simulink model "C28069_LLC_ePWM_V8_230307_PhaeShiftWorking"  (R2022b)
settings: Solver=FixedStepAuto  StartTime=0.0  StopTime=10  RelTol=1e-3  EnableMultiTasking=on
model workspace (MAT data in the model file):
  Comp_DAC = 512
undefined symbols (not defined in the file or in its folder): Down, GPTRIP1SEL, GPTRIP2SEL, PWM_Control, PWM_Gen, PWM_Gen1, SCI_A_Transmit, SCI_A_Transmit_Current_Suffix, SCI_A_Transmit_Duty_Suffix, SCI_A_Transmit_Freq_Suffix, SCI_A_Transmit_OVPFlag_Suffix, SCI_A_Transmit_PFC_Suffix, SCI_A_Transmit_SS_Suffix, SCI_A_Transmit_TBPHS_Suffix, SCI_A_Transmit_VADC_Suffix, SCI_A_Transmit_VAvg_Suffix, SCI_A_Transmit_VBAT_Suffix, SCI_A_Transmit_VBATRef_Suffix, SCI_A_Transmit_Vo_Suffix, TZ1, TZ2, u1, Up
libraries: c2802xlib x92, c280xlib x39, simulink x36, c2000lib x1
(part 4 of 18)

== system C28069_LLC_ePWM_V8_230307_PhaeShiftWorking/UART Reporting @ 1Hz/Send Current ==
  function : TriggerPort  TriggerType=function-call  VariantControl=(inherit)
  Data Store Read1 : DataStoreRead  DataStoreName=IoutCurrentBAT_Value  IndexOptions=Index vector (dialog)  Indices=1  OutputSizes=1
  Data Type Conversion : DataTypeConversion  OutDataTypeStr=double  SaturateOnIntegerOverflow=off  RndMeth=Floor
  Function Caller1 : FunctionCaller  FunctionPrototype=SCI_A_Transmit(u)  InputArgumentSpecifications=<Enter example>  OutputArgumentSpecifications=<Enter example>
  Function Caller2 : FunctionCaller  FunctionPrototype=SCI_A_Transmit_Current_Suffix()  InputArgumentSpecifications=<Enter example>  OutputArgumentSpecifications=<Enter example>
  wires:
  Data Type Conversion/1 -> Function Caller1/1
  Data Store Read1/1 -> Data Type Conversion/1

== system C28069_LLC_ePWM_V8_230307_PhaeShiftWorking/UART Reporting @ 1Hz/Send Duty ==
  function : TriggerPort  TriggerType=function-call  VariantControl=(inherit)
  Data Store Read1 : DataStoreRead  DataStoreName=Duty_Value  IndexOptions=Index vector (dialog)  Indices=1  OutputSizes=1
  Data Type Conversion : DataTypeConversion  OutDataTypeStr=double  SaturateOnIntegerOverflow=off  RndMeth=Floor
  Function Caller1 : FunctionCaller  FunctionPrototype=SCI_A_Transmit(u)  InputArgumentSpecifications=<Enter example>  OutputArgumentSpecifications=<Enter example>
  Function Caller2 : FunctionCaller  FunctionPrototype=SCI_A_Transmit_Duty_Suffix()  InputArgumentSpecifications=<Enter example>  OutputArgumentSpecifications=<Enter example>
  wires:
  Data Store Read1/1 -> Data Type Conversion/1
  Data Type Conversion/1 -> Function Caller1/1

== system C28069_LLC_ePWM_V8_230307_PhaeShiftWorking/UART Reporting @ 1Hz/Send Freq ==
  function : TriggerPort  TriggerType=function-call  VariantControl=(inherit)
  Data Store Read1 : DataStoreRead  DataStoreName=Freq_Value_Out  IndexOptions=Index vector (dialog)  Indices=1  OutputSizes=1
  Data Type Conversion : DataTypeConversion  OutDataTypeStr=double  SaturateOnIntegerOverflow=off  RndMeth=Floor
  Function Caller1 : FunctionCaller  FunctionPrototype=SCI_A_Transmit(u)  InputArgumentSpecifications=<Enter example>  OutputArgumentSpecifications=<Enter example>
  Function Caller2 : FunctionCaller  FunctionPrototype=SCI_A_Transmit_Freq_Suffix()  InputArgumentSpecifications=<Enter example>  OutputArgumentSpecifications=<Enter example>
  wires:
  Data Store Read1/1 -> Data Type Conversion/1
  Data Type Conversion/1 -> Function Caller1/1

== system C28069_LLC_ePWM_V8_230307_PhaeShiftWorking/UART Reporting @ 1Hz/Send OVPFlag ==
  function : TriggerPort  TriggerType=function-call  VariantControl=(inherit)
  Data Store Read1 : DataStoreRead  DataStoreName=OVP_Flag  IndexOptions=Index vector (dialog)  Indices=1  OutputSizes=1
  Data Type Conversion : DataTypeConversion  OutDataTypeStr=double  SaturateOnIntegerOverflow=off  RndMeth=Floor
  Function Caller1 : FunctionCaller  FunctionPrototype=SCI_A_Transmit(u)  InputArgumentSpecifications=<Enter example>  OutputArgumentSpecifications=<Enter example>
  Function Caller2 : FunctionCaller  FunctionPrototype=SCI_A_Transmit_OVPFlag_Suffix()  InputArgumentSpecifications=<Enter example>  OutputArgumentSpecifications=<Enter example>
  wires:
  Data Store Read1/1 -> Data Type Conversion/1
  Data Type Conversion/1 -> Function Caller1/1

== system C28069_LLC_ePWM_V8_230307_PhaeShiftWorking/UART Reporting @ 1Hz/Send PFC_OK ==
  function : TriggerPort  TriggerType=function-call  VariantControl=(inherit)
  Data Store Read1 : DataStoreRead  DataStoreName=PFC_OK  IndexOptions=Index vector (dialog)  Indices=1  OutputSizes=1
  Data Type Conversion : DataTypeConversion  OutDataTypeStr=double  SaturateOnIntegerOverflow=off  RndMeth=Floor
  Function Caller1 : FunctionCaller  FunctionPrototype=SCI_A_Transmit(u)  InputArgumentSpecifications=<Enter example>  OutputArgumentSpecifications=<Enter example>
  Function Caller2 : FunctionCaller  FunctionPrototype=SCI_A_Transmit_PFC_Suffix()  InputArgumentSpecifications=<Enter example>  OutputArgumentSpecifications=<Enter example>
  wires:
  Data Type Conversion/1 -> Function Caller1/1
  Data Store Read1/1 -> Data Type Conversion/1

== system C28069_LLC_ePWM_V8_230307_PhaeShiftWorking/UART Reporting @ 1Hz/Send SoftStart ==
  function : TriggerPort  TriggerType=function-call  VariantControl=(inherit)
  Data Store Read1 : DataStoreRead  DataStoreName=SoftStart_OK_Signal  IndexOptions=Index vector (dialog)  Indices=1  OutputSizes=1
  Data Type Conversion : DataTypeConversion  OutDataTypeStr=double  SaturateOnIntegerOverflow=off  RndMeth=Floor
  Function Caller1 : FunctionCaller  FunctionPrototype=SCI_A_Transmit(u)  InputArgumentSpecifications=<Enter example>  OutputArgumentSpecifications=<Enter example>
  Function Caller2 : FunctionCaller  FunctionPrototype=SCI_A_Transmit_SS_Suffix()  InputArgumentSpecifications=<Enter example>  OutputArgumentSpecifications=<Enter example>
  wires:
  Data Type Conversion/1 -> Function Caller1/1
  Data Store Read1/1 -> Data Type Conversion/1

== system C28069_LLC_ePWM_V8_230307_PhaeShiftWorking/UART Reporting @ 1Hz/Send TBPHS (PhaseShift) ==
  function : TriggerPort  TriggerType=function-call  VariantControl=(inherit)
  Data Store Read1 : DataStoreRead  DataStoreName=TBPHS  IndexOptions=Index vector (dialog)  Indices=1  OutputSizes=1
  Data Type Conversion : DataTypeConversion  OutDataTypeStr=double  SaturateOnIntegerOverflow=off  RndMeth=Floor
  Function Caller1 : FunctionCaller  FunctionPrototype=SCI_A_Transmit(u)  InputArgumentSpecifications=<Enter example>  OutputArgumentSpecifications=<Enter example>
  Function Caller2 : FunctionCaller  FunctionPrototype=SCI_A_Transmit_TBPHS_Suffix()  InputArgumentSpecifications=<Enter example>  OutputArgumentSpecifications=<Enter example>
  wires:
  Data Store Read1/1 -> Data Type Conversion/1
  Data Type Conversion/1 -> Function Caller1/1

== system C28069_LLC_ePWM_V8_230307_PhaeShiftWorking/UART Reporting @ 1Hz/Send VADC_Avg ==
  function : TriggerPort  TriggerType=function-call  VariantControl=(inherit)
  Data Store Read1 : DataStoreRead  DataStoreName=VBAT_ADC_AvgValue  IndexOptions=Index vector (dialog)  Indices=1  OutputSizes=1
  Data Type Conversion : DataTypeConversion  Commented=on  OutDataTypeStr=double  SaturateOnIntegerOverflow=off  RndMeth=Floor
  Function Caller1 : FunctionCaller  FunctionPrototype=SCI_A_Transmit(u)  InputArgumentSpecifications=<Enter example>  OutputArgumentSpecifications=<Enter example>
  Function Caller2 : FunctionCaller  FunctionPrototype=SCI_A_Transmit_VAvg_Suffix()  InputArgumentSpecifications=<Enter example>  OutputArgumentSpecifications=<Enter example>
  wires:
  Data Store Read1/1 -> Function Caller1/1

== system C28069_LLC_ePWM_V8_230307_PhaeShiftWorking/UART Reporting @ 1Hz/Send VBAT Value (Vout) ==
  function : TriggerPort  TriggerType=function-call  VariantControl=(inherit)
  Data Store Read1 : DataStoreRead  DataStoreName=VBAT_Value  IndexOptions=Index vector (dialog)  Indices=1  OutputSizes=1
  Data Type Conversion : DataTypeConversion  OutDataTypeStr=double  SaturateOnIntegerOverflow=off  RndMeth=Floor
  Function Caller1 : FunctionCaller  FunctionPrototype=SCI_A_Transmit(u)  InputArgumentSpecifications=<Enter example>  OutputArgumentSpecifications=<Enter example>
  Function Caller2 : FunctionCaller  FunctionPrototype=SCI_A_Transmit_VBAT_Suffix()  InputArgumentSpecifications=<Enter example>  OutputArgumentSpecifications=<Enter example>
  wires:
  Data Type Conversion/1 -> Function Caller1/1
  Data Store Read1/1 -> Data Type Conversion/1

== system C28069_LLC_ePWM_V8_230307_PhaeShiftWorking/UART Reporting @ 1Hz/Send VBAT Value (Vout)1 ==
  function : TriggerPort  TriggerType=function-call  VariantControl=(inherit)
  Data Store Read1 : DataStoreRead  DataStoreName=VBAT_Ref_Value  IndexOptions=Index vector (dialog)  Indices=1  OutputSizes=1
  Data Type Conversion : DataTypeConversion  OutDataTypeStr=double  SaturateOnIntegerOverflow=off  RndMeth=Floor
  Function Caller1 : FunctionCaller  FunctionPrototype=SCI_A_Transmit(u)  InputArgumentSpecifications=<Enter example>  OutputArgumentSpecifications=<Enter example>
  Function Caller2 : FunctionCaller  FunctionPrototype=SCI_A_Transmit_VBATRef_Suffix()  InputArgumentSpecifications=<Enter example>  OutputArgumentSpecifications=<Enter example>
  wires:
  Data Store Read1/1 -> Data Type Conversion/1
  Data Type Conversion/1 -> Function Caller1/1

== system C28069_LLC_ePWM_V8_230307_PhaeShiftWorking/UART Reporting @ 1Hz/Send Vo Value ==
  function : TriggerPort  TriggerType=function-call  VariantControl=(inherit)
  Data Store Read1 : DataStoreRead  DataStoreName=Vo_Value  IndexOptions=Index vector (dialog)  Indices=1  OutputSizes=1
  Data Type Conversion : DataTypeConversion  OutDataTypeStr=double  SaturateOnIntegerOverflow=off  RndMeth=Floor
  Function Caller1 : FunctionCaller  FunctionPrototype=SCI_A_Transmit(u)  InputArgumentSpecifications=<Enter example>  OutputArgumentSpecifications=<Enter example>
  Function Caller2 : FunctionCaller  FunctionPrototype=SCI_A_Transmit_Vo_Suffix()  InputArgumentSpecifications=<Enter example>  OutputArgumentSpecifications=<Enter example>
  wires:
  Data Store Read1/1 -> Data Type Conversion/1
  Data Type Conversion/1 -> Function Caller1/1

== system C28069_LLC_ePWM_V8_230307_PhaeShiftWorking/UART Reporting @ 1Hz/Send Voltage ADC Value ==
  function : TriggerPort  TriggerType=function-call  VariantControl=(inherit)
  Data Store Read1 : DataStoreRead  DataStoreName=VBAT_ADC_Value  IndexOptions=Index vector (dialog)  Indices=1  OutputSizes=1
  Data Type Conversion : DataTypeConversion  OutDataTypeStr=double  SaturateOnIntegerOverflow=off  RndMeth=Floor
  Function Caller1 : FunctionCaller  FunctionPrototype=SCI_A_Transmit(u)  InputArgumentSpecifications=<Enter example>  OutputArgumentSpecifications=<Enter example>
  Function Caller2 : FunctionCaller  FunctionPrototype=SCI_A_Transmit_VADC_Suffix()  InputArgumentSpecifications=<Enter example>  OutputArgumentSpecifications=<Enter example>
  wires:
  Data Store Read1/1 -> Data Type Conversion/1
  Data Type Conversion/1 -> Function Caller1/1

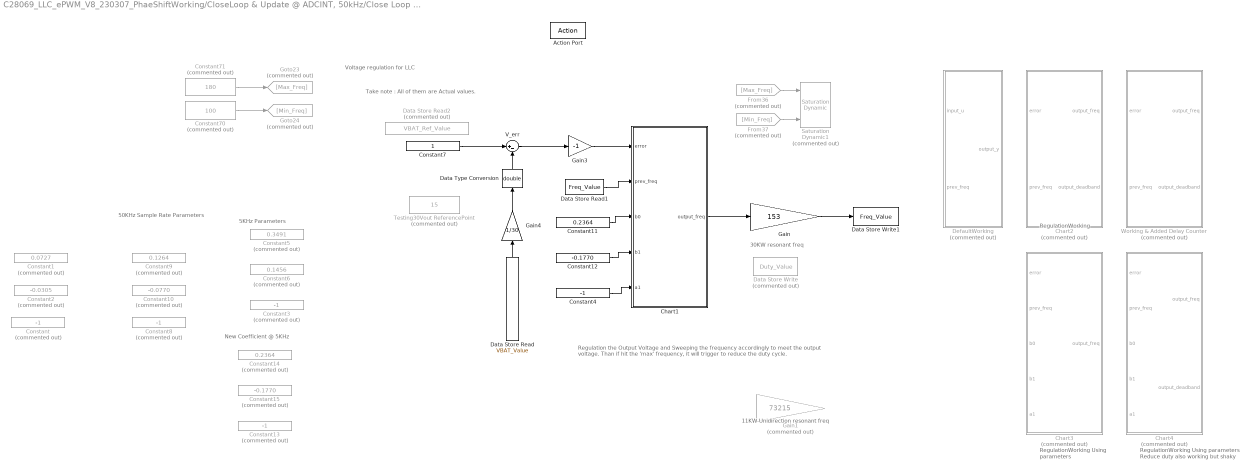
== system C28069_LLC_ePWM_V8_230307_PhaeShiftWorking/CloseLoop & Update @ ADCINT, 50kHz/Close Loop Regulation1/If Action Subsystem ==
  note: New Coefficient @ 5KHz
  note: 50KHz Sample Rate
      | Parameters
  note: RegulationWorking
  note: Regulation the Output Voltage and Sweeping the frequency accordingly to meet the output voltage.
      | Than if hit the 'max' frequency, it will trigger to reduce the duty cycle.
  note: Voltage regulation for LLC
  note: Take note : All of them are Actual values.
  note: 11KW Unidirection resonant freq
  note: 30KW resonant freq
  note: 5KHz Parameters
  note: RegulationWorking
      | Using parameters
  note: RegulationWorking
      | Using parameters
      | Reduce duty also working but shaky
  Action Port : ActionPort  ActionPortLabel=if((u1 == 1) & (u2 == 1))
  Chart1 : Stateflow chart  TreatAsAtomicUnit=on
  Chart2 : Stateflow chart  Commented=on  TreatAsAtomicUnit=on
  Chart3 : Stateflow chart  Commented=on  TreatAsAtomicUnit=on
  Chart4 : Stateflow chart  Commented=on  TreatAsAtomicUnit=on
  Constant{,3,8,13} (4 alike) : Constant  Commented=on  Value=-1  OutDataTypeStr=double
  Constant1 : Constant  Commented=on  Value=0.0727  OutDataTypeStr=double
  Constant10 : Constant  Commented=on  Value=-0.0770  OutDataTypeStr=double
  Constant11 : Constant  Value=0.2364  OutDataTypeStr=double
  Constant12 : Constant  Value=-0.1770  OutDataTypeStr=double
  Constant14 : Constant  Commented=on  Value=0.2364  OutDataTypeStr=double
  Constant15 : Constant  Commented=on  Value=-0.1770  OutDataTypeStr=double
  Constant2 : Constant  Commented=on  Value=-0.0305  OutDataTypeStr=double
  Constant4 : Constant  Value=-1  OutDataTypeStr=double
  Constant5 : Constant  Commented=on  Value=0.3491  OutDataTypeStr=double
  Constant6 : Constant  Commented=on  Value=0.1456  OutDataTypeStr=double
  Constant7 : Constant  OutDataTypeStr=double
  Constant70 : Constant  Commented=on  Value=100  OutDataTypeStr=double
  Constant71 : Constant  Commented=on  Value=180  OutDataTypeStr=double
  Constant9 : Constant  Commented=on  Value=0.1264  OutDataTypeStr=double
  Data Store Read : DataStoreRead  DataStoreName=VBAT_Value  IndexOptions=Index vector (dialog)  Indices=1  OutputSizes=1
  Data Store Read1 : DataStoreRead  DataStoreName=Freq_Value  IndexOptions=Index vector (dialog)  Indices=1  OutputSizes=1
  Data Store Read2 : DataStoreRead  Commented=on  DataStoreName=VBAT_Ref_Value  IndexOptions=Index vector (dialog)  Indices=1  OutputSizes=1
  Data Store Write : DataStoreWrite  Commented=on  DataStoreName=Duty_Value  IndexOptions=Index vector (dialog)  Indices=1  OutputSizes=1
  Data Store Write1 : DataStoreWrite  DataStoreName=Freq_Value  IndexOptions=Index vector (dialog)  Indices=1  OutputSizes=1
  Data Type Conversion : DataTypeConversion  OutDataTypeStr=double  SaturateOnIntegerOverflow=off  RndMeth=Floor
  DefaultWorking : Stateflow chart  Commented=on  TreatAsAtomicUnit=on
  From36 : From  Commented=on  GotoTag=Max_Freq
  From37 : From  Commented=on  GotoTag=Min_Freq
  Gain : Gain  Gain=153
  Gain1 : Gain  Commented=on  Gain=73215
  Gain3 : Gain  Gain=-1
  Gain4 : Gain  Gain=1/30
  Goto23 : Goto  Commented=on  GotoTag=Max_Freq
  Goto24 : Goto  Commented=on  GotoTag=Min_Freq
  Saturation Dynamic1 : simulink/Discontinuities/Saturation Dynamic  Commented=on  OutMin=[]  OutMax=[]  OutDataTypeStr=double  OutputDataTypeScalingMode=single  OutDataType=single  OutScaling=2^-10  DoSatur=off
  Testing30Vout ReferencePoint : Constant  Commented=on  Value=15  OutDataTypeStr=double
  V_err : Sum  Inputs=|+-  AccumDataTypeStr=double  OutDataTypeStr=double
  Working & Added Delay Counter : Stateflow chart  Commented=on  TreatAsAtomicUnit=on
  wires:
  Data Type Conversion/1 -> V_err/2
  Data Store Read1/1 -> Chart1/2(prev_freq)
  Constant70/1 -> Goto24/1
  From37/1 -> Saturation Dynamic1/3
  From36/1 -> Saturation Dynamic1/1
  V_err/1 -> Gain3/1
  Constant71/1 -> Goto23/1
  Chart1/1(output_freq) -> Gain/1
  Gain/1 -> Data Store Write1/1
  Data Store Read/1 -> Gain4/1
  Gain3/1 -> Chart1/1(error)
  Gain4/1 -> Data Type Conversion/1
  Constant11/1 -> Chart1/3(b0)
  Constant12/1 -> Chart1/4(b1)
  Constant4/1 -> Chart1/5(a1)
  Constant7/1 -> V_err/1

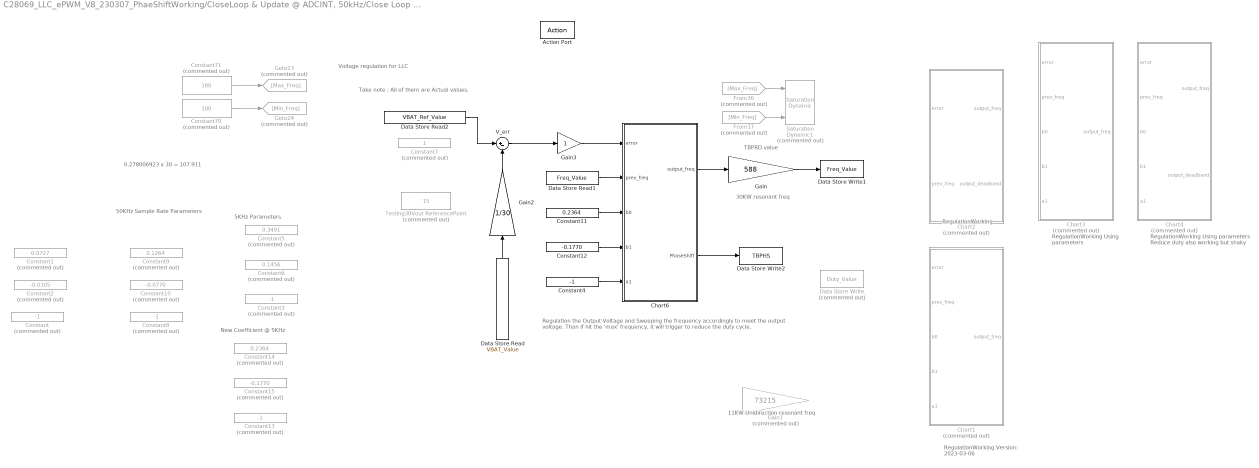
== system C28069_LLC_ePWM_V8_230307_PhaeShiftWorking/CloseLoop & Update @ ADCINT, 50kHz/Close Loop Regulation2/If Action Subsystem ==
  note: 0.278006923 x 30 = 107.911
  note: New Coefficient @ 5KHz
  note: 50KHz Sample Rate
      | Parameters
  note: RegulationWorking
  note: Regulation the Output Voltage and Sweeping the frequency accordingly to meet the output voltage.
      | Than if hit the 'max' frequency, it will trigger to reduce the duty cycle.
  note: Voltage regulation for LLC
  note: Take note : All of them are Actual values.
  note: 11KW Unidirection resonant freq
  note: 30KW resonant freq
  note: 5KHz Parameters
  note: RegulationWorking
      | Using parameters
  note: RegulationWorking
      | Using parameters
      | Reduce duty also working but shaky
  note: TBPRD value
  note: RegulationWorking
      | Version: 2023-03-06
  Action Port : ActionPort  ActionPortLabel=if((u1 == 1))
  Chart1 : Stateflow chart  Commented=on  TreatAsAtomicUnit=on
  Chart2 : Stateflow chart  Commented=on  TreatAsAtomicUnit=on
  Chart3 : Stateflow chart  Commented=on  TreatAsAtomicUnit=on
  Chart4 : Stateflow chart  Commented=on  TreatAsAtomicUnit=on
  Chart6 : Stateflow chart  TreatAsAtomicUnit=on
  Constant{,3,8,13} (4 alike) : Constant  Commented=on  Value=-1  OutDataTypeStr=double
  Constant1 : Constant  Commented=on  Value=0.0727  OutDataTypeStr=double
  Constant10 : Constant  Commented=on  Value=-0.0770  OutDataTypeStr=double
  Constant11 : Constant  Value=0.2364  OutDataTypeStr=double
  Constant12 : Constant  Value=-0.1770  OutDataTypeStr=double
  Constant14 : Constant  Commented=on  Value=0.2364  OutDataTypeStr=double
  Constant15 : Constant  Commented=on  Value=-0.1770  OutDataTypeStr=double
  Constant2 : Constant  Commented=on  Value=-0.0305  OutDataTypeStr=double
  Constant4 : Constant  Value=-1  OutDataTypeStr=double
  Constant5 : Constant  Commented=on  Value=0.3491  OutDataTypeStr=double
  Constant6 : Constant  Commented=on  Value=0.1456  OutDataTypeStr=double
  Constant7 : Constant  Commented=on  OutDataTypeStr=double
  Constant70 : Constant  Commented=on  Value=100  OutDataTypeStr=double
  Constant71 : Constant  Commented=on  Value=180  OutDataTypeStr=double
  Constant9 : Constant  Commented=on  Value=0.1264  OutDataTypeStr=double
  Data Store Read : DataStoreRead  DataStoreName=VBAT_Value  IndexOptions=Index vector (dialog)  Indices=1  OutputSizes=1
  Data Store Read1 : DataStoreRead  DataStoreName=Freq_Value  IndexOptions=Index vector (dialog)  Indices=1  OutputSizes=1
  Data Store Read2 : DataStoreRead  DataStoreName=VBAT_Ref_Value  IndexOptions=Index vector (dialog)  Indices=1  OutputSizes=1
  Data Store Write : DataStoreWrite  Commented=on  DataStoreName=Duty_Value  IndexOptions=Index vector (dialog)  Indices=1  OutputSizes=1
  Data Store Write1 : DataStoreWrite  DataStoreName=Freq_Value  IndexOptions=Index vector (dialog)  Indices=1  OutputSizes=1
  Data Store Write2 : DataStoreWrite  DataStoreName=TBPHS  IndexOptions=Index vector (dialog)  Indices=1  OutputSizes=1
  From36 : From  Commented=on  GotoTag=Max_Freq
  From37 : From  Commented=on  GotoTag=Min_Freq
  Gain : Gain  Gain=588
  Gain1 : Gain  Commented=on  Gain=73215
  Gain2 : Gain  Gain=1/30
  Gain3 : Gain
  Goto23 : Goto  Commented=on  GotoTag=Max_Freq
  Goto24 : Goto  Commented=on  GotoTag=Min_Freq
  Saturation Dynamic1 : simulink/Discontinuities/Saturation Dynamic  Commented=on  OutMin=[]  OutMax=[]  OutDataTypeStr=double  OutputDataTypeScalingMode=single  OutDataType=single  OutScaling=2^-10  DoSatur=off
  Testing30Vout ReferencePoint : Constant  Commented=on  Value=15  OutDataTypeStr=double
  V_err : Sum  Inputs=|+-  AccumDataTypeStr=double  OutDataTypeStr=double
  wires:
  Data Store Read1/1 -> Chart6/2(prev_freq)
  Constant70/1 -> Goto24/1
  From37/1 -> Saturation Dynamic1/3
  From36/1 -> Saturation Dynamic1/1
  V_err/1 -> Gain3/1
  Constant71/1 -> Goto23/1
  Gain/1 -> Data Store Write1/1
  Gain3/1 -> Chart6/1(error)
  Constant11/1 -> Chart6/3(b0)
  Constant12/1 -> Chart6/4(b1)
  Constant4/1 -> Chart6/5(a1)
  Data Store Read/1 -> Gain2/1
  Gain2/1 -> V_err/2
  Data Store Read2/1 -> V_err/1
  Chart6/1(output_freq) -> Gain/1
  Chart6/2(PhaseShift) -> Data Store Write2/1

== system C28069_LLC_ePWM_V8_230307_PhaeShiftWorking/CloseLoop & Update @ ADCINT, 50kHz/Control/Close Loop Regulation ==
  function : TriggerPort  TriggerType=function-call  VariantControl=(inherit)
  Constant : Constant
  Data Store Read1 : DataStoreRead  DataStoreName=SoftStart_OK_Signal  IndexOptions=Index vector (dialog)  Indices=1  OutputSizes=1
  Data Store Read4 : DataStoreRead  DataStoreName=PFC_OK  IndexOptions=Index vector (dialog)  Indices=1  OutputSizes=1
  If : If  NumInputs=2  IfExpression=(u1 == 1) & (u2 == 1)  ShowElse=off
  If Action Subsystem : Subsystem  TreatAsAtomicUnit=on
  wires:
  Constant/1 -> If/2
  If/1 -> If Action Subsystem/Action
  Data Store Read4/1 -> If/1

== system C28069_LLC_ePWM_V8_230307_PhaeShiftWorking/CloseLoop & Update @ ADCINT, 50kHz/Control/Debug ==
  function : TriggerPort  TriggerType=function-call  VariantControl=(inherit)
  Constant3 : Constant
  GPIO21 : c280xlib/Digital Output  GPIO_Number=GPIO16~GPIO23  GPIO_Bit0=off  GPIO_BIT0_Toggle=off  GPIO_Bit1=off  GPIO_BIT1_Toggle=off  GPIO_Bit2=off  GPIO_BIT2_Toggle=off  GPIO_Bit3=off  GPIO_BIT3_Toggle=off  GPIO_Bit4=off  GPIO_BIT4_Toggle=off  GPIO_Bit5=on  GPIO_BIT5_Toggle=off  GPIO_Bit6=off  GPIO_BIT6_Toggle=off  GPIO_Bit7=off  GPIO_BIT7_Toggle=off
  wires:
  Constant3/1 -> GPIO21/1

== system C28069_LLC_ePWM_V8_230307_PhaeShiftWorking/CloseLoop & Update @ ADCINT, 50kHz/Control/Debug1 ==
  function : TriggerPort  TriggerType=function-call  VariantControl=(inherit)
  Constant3 : Constant  Value=0
  GPIO21 : c280xlib/Digital Output  GPIO_Number=GPIO16~GPIO23  GPIO_Bit0=off  GPIO_BIT0_Toggle=off  GPIO_Bit1=off  GPIO_BIT1_Toggle=off  GPIO_Bit2=off  GPIO_BIT2_Toggle=off  GPIO_Bit3=off  GPIO_BIT3_Toggle=off  GPIO_Bit4=off  GPIO_BIT4_Toggle=off  GPIO_Bit5=on  GPIO_BIT5_Toggle=off  GPIO_Bit6=off  GPIO_BIT6_Toggle=off  GPIO_Bit7=off  GPIO_BIT7_Toggle=off
  wires:
  Constant3/1 -> GPIO21/1

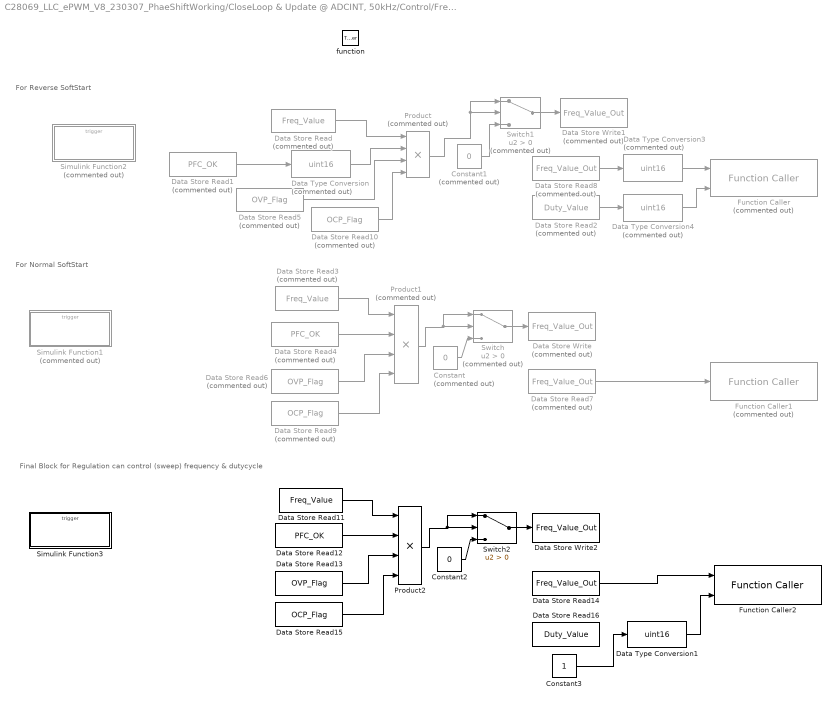
== system C28069_LLC_ePWM_V8_230307_PhaeShiftWorking/CloseLoop & Update @ ADCINT, 50kHz/Control/Frequency Update ==
  note: For Reverse SoftStart
  note: For Normal SoftStart
  note: Final Block for Regulation can control (sweep) frequency & dutycycle
  function : TriggerPort  TriggerType=function-call  VariantControl=(inherit)
  Constant : Constant  Commented=on  Value=0  OutDataTypeStr=double
  Constant1 : Constant  Commented=on  Value=0
  Constant2 : Constant  Value=0  OutDataTypeStr=double
  Constant3 : Constant  OutDataTypeStr=double
  Data Store Read : DataStoreRead  Commented=on  DataStoreName=Freq_Value  IndexOptions=Index vector (dialog)  Indices=1  OutputSizes=1
  Data Store Read1 : DataStoreRead  Commented=on  DataStoreName=PFC_OK  IndexOptions=Index vector (dialog)  Indices=1  OutputSizes=1
  Data Store Read10 : DataStoreRead  Commented=on  DataStoreName=OCP_Flag  IndexOptions=Index vector (dialog)  Indices=1  OutputSizes=1
  Data Store Read11 : DataStoreRead  DataStoreName=Freq_Value  IndexOptions=Index vector (dialog)  Indices=1  OutputSizes=1
  Data Store Read12 : DataStoreRead  DataStoreName=PFC_OK  IndexOptions=Index vector (dialog)  Indices=1  OutputSizes=1
  Data Store Read13 : DataStoreRead  DataStoreName=OVP_Flag  IndexOptions=Index vector (dialog)  Indices=1  OutputSizes=1
  Data Store Read14 : DataStoreRead  DataStoreName=Freq_Value_Out  IndexOptions=Index vector (dialog)  Indices=1  OutputSizes=1
  Data Store Read15 : DataStoreRead  DataStoreName=OCP_Flag  IndexOptions=Index vector (dialog)  Indices=1  OutputSizes=1
  Data Store Read16 : DataStoreRead  DataStoreName=Duty_Value  IndexOptions=Index vector (dialog)  Indices=1  OutputSizes=1
  Data Store Read2 : DataStoreRead  Commented=on  DataStoreName=Duty_Value  IndexOptions=Index vector (dialog)  Indices=1  OutputSizes=1
  Data Store Read3 : DataStoreRead  Commented=on  DataStoreName=Freq_Value  IndexOptions=Index vector (dialog)  Indices=1  OutputSizes=1
  Data Store Read4 : DataStoreRead  Commented=on  DataStoreName=PFC_OK  IndexOptions=Index vector (dialog)  Indices=1  OutputSizes=1
  Data Store Read5 : DataStoreRead  Commented=on  DataStoreName=OVP_Flag  IndexOptions=Index vector (dialog)  Indices=1  OutputSizes=1
  Data Store Read6 : DataStoreRead  Commented=on  DataStoreName=OVP_Flag  IndexOptions=Index vector (dialog)  Indices=1  OutputSizes=1
  Data Store Read7 : DataStoreRead  Commented=on  DataStoreName=Freq_Value_Out  IndexOptions=Index vector (dialog)  Indices=1  OutputSizes=1
  Data Store Read8 : DataStoreRead  Commented=on  DataStoreName=Freq_Value_Out  IndexOptions=Index vector (dialog)  Indices=1  OutputSizes=1
  Data Store Read9 : DataStoreRead  Commented=on  DataStoreName=OCP_Flag  IndexOptions=Index vector (dialog)  Indices=1  OutputSizes=1
  Data Store Write : DataStoreWrite  Commented=on  DataStoreName=Freq_Value_Out  IndexOptions=Index vector (dialog)  Indices=1  OutputSizes=1
  Data Store Write1 : DataStoreWrite  Commented=on  DataStoreName=Freq_Value_Out  IndexOptions=Index vector (dialog)  Indices=1  OutputSizes=1
  Data Store Write2 : DataStoreWrite  DataStoreName=Freq_Value_Out  IndexOptions=Index vector (dialog)  Indices=1  OutputSizes=1
  Data Type Conversion : DataTypeConversion  Commented=on  OutDataTypeStr=uint16  SaturateOnIntegerOverflow=off  RndMeth=Floor
  Data Type Conversion1 : DataTypeConversion  OutDataTypeStr=uint16  SaturateOnIntegerOverflow=off  RndMeth=Floor
  Data Type Conversion3 : DataTypeConversion  Commented=on  OutDataTypeStr=uint16  SaturateOnIntegerOverflow=off  RndMeth=Floor
  Data Type Conversion4 : DataTypeConversion  Commented=on  OutDataTypeStr=uint16  SaturateOnIntegerOverflow=off  RndMeth=Floor
  Function Caller : FunctionCaller  Commented=on  FunctionPrototype=PWM_Gen1(u,u1)  InputArgumentSpecifications=<Enter example>  OutputArgumentSpecifications=<Enter example>
  Function Caller1 : FunctionCaller  Commented=on  FunctionPrototype=PWM_Gen(u)  InputArgumentSpecifications=<Enter example>  OutputArgumentSpecifications=<Enter example>
  Function Caller2 : FunctionCaller  FunctionPrototype=PWM_Control(u,u1)  InputArgumentSpecifications=<Enter example>  OutputArgumentSpecifications=<Enter example>
  Product : Product  Commented=on  Inputs=4  OutDataTypeStr=uint16
  Product1 : Product  Commented=on  Inputs=4  OutDataTypeStr=double
  Product2 : Product  Inputs=4  OutDataTypeStr=double
  Simulink Function1 : Subsystem  Commented=on  TreatAsAtomicUnit=on
  Simulink Function2 : Subsystem  Commented=on  TreatAsAtomicUnit=on
  Simulink Function3 : Subsystem  TreatAsAtomicUnit=on
  Switch : Switch  Commented=on  Criteria=u2 > Threshold  OutDataTypeStr=double  SaturateOnIntegerOverflow=off  InputSameDT=off
  Switch1 : Switch  Commented=on  Criteria=u2 > Threshold  SaturateOnIntegerOverflow=off  InputSameDT=off
  Switch2 : Switch  Criteria=u2 > Threshold  OutDataTypeStr=double  SaturateOnIntegerOverflow=off  InputSameDT=off
  wires:
  Data Store Read1/1 -> Data Type Conversion/1
  Data Type Conversion/1 -> Product/2
  Data Store Read7/1 -> Function Caller1/1
  Product1/1 -> Switch/2, Switch/1
  Data Store Read2/1 -> Data Type Conversion4/1
  Data Store Read10/1 -> Product/4
  Data Store Read5/1 -> Product/3
  Constant1/1 -> Switch1/3
  Data Store Read4/1 -> Product1/2
  Data Store Read/1 -> Product/1
  Product/1 -> Switch1/2, Switch1/1
  Data Store Read9/1 -> Product1/4
  Constant/1 -> Switch/3
  Data Type Conversion3/1 -> Function Caller/1
  Data Store Read6/1 -> Product1/3
  Switch1/1 -> Data Store Write1/1
  Switch/1 -> Data Store Write/1
  Data Type Conversion4/1 -> Function Caller/2
  Data Store Read3/1 -> Product1/1
  Data Store Read8/1 -> Data Type Conversion3/1
  Constant2/1 -> Switch2/3
  Data Store Read11/1 -> Product2/1
  Switch2/1 -> Data Store Write2/1
  Data Store Read15/1 -> Product2/4
  Data Store Read13/1 -> Product2/3
  Product2/1 -> Switch2/2, Switch2/1
  Data Store Read12/1 -> Product2/2
  Data Store Read14/1 -> Function Caller2/1
  Data Type Conversion1/1 -> Function Caller2/2
  Constant3/1 -> Data Type Conversion1/1

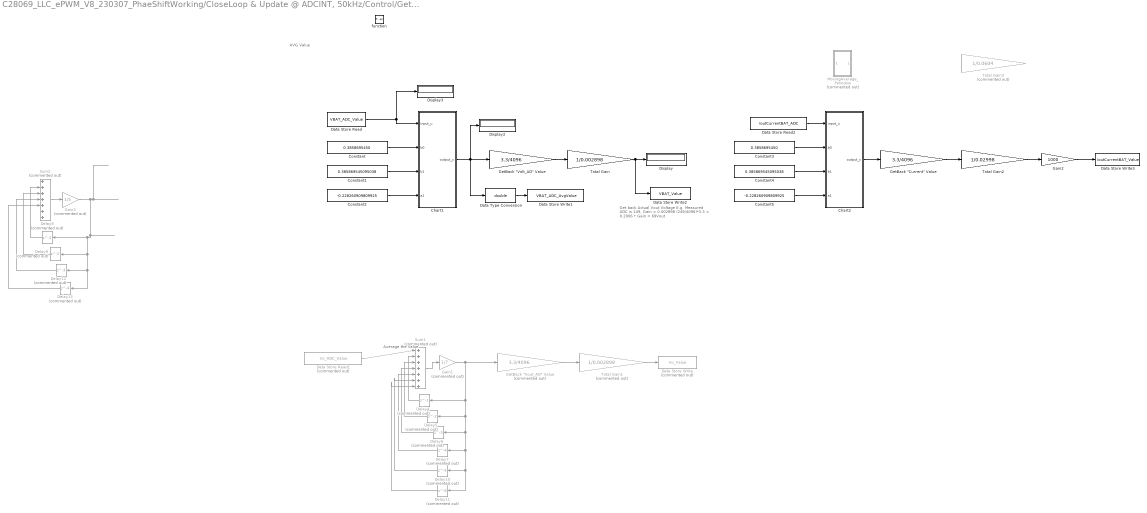
== system C28069_LLC_ePWM_V8_230307_PhaeShiftWorking/CloseLoop & Update @ ADCINT, 50kHz/Control/Get AVG2 ==
  note: AVG Value
  note: Average the value
  note: Get back Actual Vout Voltage
      | E.g.
      | Measured ADC is 249, Gain = 0.002898
      | (249/4096)*3.3 = 0.2006 * Gain
      | = 69Vout
  function : TriggerPort  TriggerType=function-call  VariantControl=(inherit)
  Chart1 : Stateflow chart  TreatAsAtomicUnit=on
  Chart2 : Stateflow chart  TreatAsAtomicUnit=on
  Constant : Constant  Value=0.3858695450
  Constant1 : Constant  Value=0.385869545095038
  Constant2 : Constant  Value=-0.228260909809925
  Constant3 : Constant  Value=0.3858695450
  Constant4 : Constant  Value=0.385869545095038
  Constant5 : Constant  Value=-0.228260909809925
  Data Store Read : DataStoreRead  DataStoreName=VBAT_ADC_Value  IndexOptions=Index vector (dialog)  Indices=1  OutputSizes=1
  Data Store Read1 : DataStoreRead  Commented=on  DataStoreName=Vo_ADC_Value  IndexOptions=Index vector (dialog)  Indices=1  OutputSizes=1
  Data Store Read2 : DataStoreRead  DataStoreName=IoutCurrentBAT_ADC  IndexOptions=Index vector (dialog)  Indices=1  OutputSizes=1
  Data Store Write : DataStoreWrite  Commented=on  DataStoreName=Vo_Value  IndexOptions=Index vector (dialog)  Indices=1  OutputSizes=1
  Data Store Write1 : DataStoreWrite  DataStoreName=VBAT_ADC_AvgValue  IndexOptions=Index vector (dialog)  Indices=1  OutputSizes=1
  Data Store Write2 : DataStoreWrite  DataStoreName=VBAT_Value  IndexOptions=Index vector (dialog)  Indices=1  OutputSizes=1
  Data Store Write3 : DataStoreWrite  DataStoreName=IoutCurrentBAT_Value  IndexOptions=Index vector (dialog)  Indices=1  OutputSizes=1
  Data Type Conversion : DataTypeConversion  OutDataTypeStr=double  SaturateOnIntegerOverflow=off  RndMeth=Floor
  Delay10 : Delay  Commented=on  DelayLength=5
  Delay11 : Delay  Commented=on  DelayLength=6
  Delay12 : Delay  Commented=on  DelayLength=3
  Delay13 : Delay  Commented=on  DelayLength=4
  Delay4 : Delay  Commented=on  DelayLength=1
  Delay5 : Delay  Commented=on
  Delay6 : Delay  Commented=on  DelayLength=3
  Delay7 : Delay  Commented=on  DelayLength=4
  Delay8 : Delay  Commented=on  DelayLength=1
  Delay9 : Delay  Commented=on
  Display : Display
      settings: Decimation=2
  Display2 : Display
  Display3 : Display
  Gain1 : Gain  Commented=on  Gain=1/7  OutDataTypeStr=uint16
  Gain2 : Gain  Gain=1000
  Gain3 : Gain  Commented=on  Gain=1/5  OutDataTypeStr=uint16
  "GetBack \"Current\" Value" : Gain  Gain=3.3/4096  OutDataTypeStr=double
  "GetBack \"Volt_AD\" Value" : Gain  Gain=3.3/4096  OutDataTypeStr=double
  "GetBack \"Vout_AD\" Value" : Gain  Commented=on  Gain=3.3/4096  OutDataTypeStr=double
  MovingAverage_7Window : Subsystem  Commented=on
  Sum1 : Sum  Commented=on  Inputs=|+++++++
  Sum2 : Sum  Commented=on  Inputs=|+++++++
  Total Gain : Gain  Gain=1/0.002898  OutDataTypeStr=double
  Total Gain1 : Gain  Commented=on  Gain=1/0.002898  OutDataTypeStr=double
  Total Gain2 : Gain  Gain=1/0.02998  OutDataTypeStr=double
  Total Gain3 : Gain  Commented=on  Gain=1/0.0604  OutDataTypeStr=double
  wires:
  Delay4/1 -> Sum1/2
  Total Gain1/1 -> Data Store Write/1
  "GetBack \"Current\" Value"/1 -> Total Gain2/1
  Delay7/1 -> Sum1/5
  Gain1/1 -> Delay4/1, Delay5/1, Delay6/1, Delay7/1, Delay10/1, Delay11/1, "GetBack \"Vout_AD\" Value"/1
  Data Type Conversion/1 -> Data Store Write1/1
  Delay6/1 -> Sum1/4
  Delay11/1 -> Sum1/7
  Delay10/1 -> Sum1/6
  "GetBack \"Vout_AD\" Value"/1 -> Total Gain1/1
  "GetBack \"Volt_AD\" Value"/1 -> Total Gain/1
  Data Store Read1/1 -> Sum1/1
  Total Gain/1 -> Display/1, Data Store Write2/1
  Sum1/1 -> Gain1/1
  Delay5/1 -> Sum1/3
  Total Gain2/1 -> Gain2/1
  Gain2/1 -> Data Store Write3/1
  Gain3/1 -> Delay9/1, Delay12/1, Delay13/1, Delay8/1
  Delay9/1 -> Sum2/3
  Sum2/1 -> Gain3/1
  Delay13/1 -> Sum2/5
  Delay12/1 -> Sum2/4
  Delay8/1 -> Sum2/2
  Data Store Read/1 -> Chart1/1(input_u), Display3/1
  Constant2/1 -> Chart1/4(a1)
  Constant1/1 -> Chart1/3(b1)
  Constant/1 -> Chart1/2(b0)
  Chart1/1(output_y) -> Display2/1, Data Type Conversion/1, "GetBack \"Volt_AD\" Value"/1
  Constant3/1 -> Chart2/2(b0)
  Constant4/1 -> Chart2/3(b1)
  Constant5/1 -> Chart2/4(a1)
  Data Store Read2/1 -> Chart2/1(input_u)
  Chart2/1(output_y) -> "GetBack \"Current\" Value"/1

== system C28069_LLC_ePWM_V8_230307_PhaeShiftWorking/CloseLoop & Update @ ADCINT, 50kHz/Frequency Update/Simulink Function1 ==
  note: Original
  note: Frequency Input Selection
  note: Control CMPA/B to Zero
      | When the input is <1KHz
      | (To switch off ePWM)
  note: Fixing deadtime to 250ns
  note: Added Trigger
  note: For F28069M
  PWM_Control2 : TriggerPort  TriggerType=function-call  IsSimulinkFunction=on  FunctionName=PWM_Control2  FunctionVisibility=scoped  VariantControl=(inherit)
  CMPA : Display
  CMPA1 : Display
  CMPB : Display
  CMPB1 : Display
  Constant : Constant  Value=100
  Constant1 : Constant
  Constant2 : Constant  Value=0
  Constant3 : Constant  Commented=on  Value=50
  Constant4 : Constant
  Dead time (%) : Display
  Dead time (sec) : Constant  Value=250E-9
  Divide : Product  Inputs=*/
  Floor : Rounding
  Gain : Gain  Gain=1/45000
  Gain1 : Gain  Gain=1000
  Gain2 : Gain  Gain=100
  Product1 : Product  Inputs=3
  Product2 : Product
  Product3 : Product
  Product4 : Product
  Subsystem1 : Subsystem  Commented=on
  Subtract : Sum  Inputs=+-
  Switch : Switch  Criteria=u2 > Threshold  Threshold=1  SaturateOnIntegerOverflow=off  InputSameDT=off
  Switch1 : Switch  Criteria=u2 > Threshold  OutDataTypeStr=double  SaturateOnIntegerOverflow=off  InputSameDT=off
  ePWM1 : c2802xlib/ePWM  PwmType=C2000  useModule=ePWM6  ePWMxLINKTBPRD=Not Linked  periodUnits=Clock cycles  timerSource=Input port  timerPeriod_clk=294  timerPeriod_sec=0.0001  tbshadow=Counter equals to zero  countingMode=Up-Down  phaseActiveEnable=Disable  phaseDirection=Count down after sync  phaseActive=0  synchronizationEnable=off  dcaevt1Sync=off  dcbevt1Sync=off  synchronizationOption=Disable  dcbevt1SyncOut=off  dcaevt1SyncOut=off  cmpdSyncOut=off  cmpcSyncOut=off  cmpbSyncOut=off  zeroSyncOut=off  swfSyncOut=off  perSynchronizationOption=Counter equals to period (CTR=PRD)  clockPrescale=1  HSclockPrescale=1  enswap=off  ePWMxAStatus=on  ePWMxAactionLogic1=Do nothing  ePWMxAactionLogic2=Do nothing  ePWMxAactionLogic3=Set  ePWMxAactionLogic4=Do nothing  ePWMxAactionLogic5=Clear  ePWMxAactionLogic6=Do nothing  ePWMxACSFenable=off  ePWMxACSFvalue=Forcing disable  ePWMxASFreload=Zero  ePWMxBStatus=on  ePWMxBactionLogic1=Do nothing  ePWMxBactionLogic2=Do nothing  ePWMxBactionLogic3=Do nothing  ePWMxBactionLogic4=Clear  ePWMxBactionLogic5=Do nothing  ePWMxBactionLogic6=Set  ePWMxBCSFenable=off  ePWMxBCSFvalue=Forcing disable  ePWMxBSFreload=Zero  ePWNxBOutWay=off  ePWMxLINKCMPA=Not Linked  CMPAUnits=Clock cycles  CMPASource=Input port  CMPAValue_per=50  CMPAValue_clk=0  enCMPAshadow=Counter equals to zero (CTR=Zero)  ePWMxLINKCMPB=Not Linked  CMPBUnits=Clock cycles  CMPBSource=Input port  CMPBValue_per=50  CMPBValue_clk=0  enCMPBshadow=Counter equals to zero (CTR=Zero)  ePWMxLINKCMPC=Not Linked  CMPCUnits=Clock cycles  CMPCSource=Specify via dialog  CMPCValue_per=50  CMPCValue_clk=32000  enCMPCshadow=Counter equals to zero (CTR=Zero)  ePWMxLINKCMPD=Not Linked  CMPDUnits=Clock cycles  CMPDSource=Specify via dialog  CMPDValue_per=50  CMPDValue_clk=32000  enCMPDshadow=Counter equals to zero (CTR=Zero)  enableDBePWMxA=off  enableDBePWMxB=off  enhalfcycle=off  DBpolarity=Active high complementary (AHC)  DBedgeDelay=Positive  DBSource_ePWMxA=ePWMxA  DBSource_ePWMxB=ePWMxA  DBPeriodUnits=Clock cycles  DBperiodSource=Input port  REDperiod=10  FEDperiod=10  REDperiod_sec=0  FEDperiod_sec=0  LoadModeDBRED=Immediate without using shadow  LoadModeDBFED=Immediate without using shadow  adcstartModuleA=off  adcrequestEventA=First event  adcstartEventA=Counter equals to zero (CTR=Zero)  adcstartEventA_type2=Digital Compare Module A Event 1 start of conversion (DCAEVT1.soc)  adcstartModuleB=off  adcrequestEventB=First event  adcstartEventB=Counter equals to zero (CTR=Zero)  adcstartEventB_type2=Counter equals to zero (CTR=Zero)  intEn=off  intPrd=First event  intSel=Counter equals to zero (CTR=Zero)  intSel_type2=Counter equals to zero (CTR=Zero)  hrpe=off  enHRPWM=off  HRPWM_LoadMode=Counter equals to period (CTR=PRD)  HRPWM_CTLMode=Duty or Period control mode  HRPWM_EDGMode=Both edge  hrpeb=off  enHRPWMB=off  HRPWM_LoadModeB=Counter equals to zero (CTR=ZERO)  HRPWM_CTLModeB=Duty or Period control mode  HRPWM_EDGModeB=Both edge  enHRDBRED=off  enHRDBFED=off  enSFO=on  enautoconv=on  chopperEnable=off  chopperFrequency=1  chopperFirstwidth=1  chopperDuty=12.5%  tripZonesource=Specify via dialog  tzselOSHT1=off  tzselOSHT2=off  tzselOSHT3=off  tzselOSHDCAEV1=off  tzselOSHDCBEV1=off  tzselCBC1=off  tzselCBC2=off  tzselCBC3=off  tzselCBCDCAEV2=off  tzselCBCDCBEV2=off  tzselOSHT4=off  tzselOSHT5=off  tzselOSHT6=off  tzselCBC4=off  tzselCBC5=off  tzselCBC6=off  enTzOstIntr=off  enTzCbcIntr=off  enTzDCAEVT1Intr=off  enTzDCAEVT2Intr=off  enTzDCBEVT1Intr=off  enTzDCBEVT2Intr=off  ePWMxAforced=No action  ePWMxBforced=No action  DCAEVT1forced=Low  DCBEVT1forced=Low  DCAEVT2forced=No action  DCBEVT2forced=No action  dcah=COMP1OUT input  dcal=Trip Zone 1 input (TZ1)  dcbh=COMP1OUT input  dcbl=Trip Zone 1 input (TZ1)  dcah_type2=GPTRIP1SEL/(TZ1)  dcal_type2=GPTRIP2SEL/(TZ2)  dcbh_type2=GPTRIP1SEL/(TZ1)  dcbl_type2=GPTRIP2SEL/(TZ2)  gendcaevt1=DCAH=high and DCAL=don't care  gendcaevt2=Event disabled  gendcbevt1=DCBH=high and DCBL=don't care  gendcbevt2=Event disabled  dcaevt1src=DCAEVT1 with sync  dcaevt2src=DCAEVT2 with sync  dcbevt1src=DCBEVT1 with sync  dcbevt2src=DCBEVT2 with sync  pulsesel=Counter equals to zero (CTR=Zero)  blankinv=off  blankoffset=0  blankwidth=0  evsrcsel=Filtered version of DCAEVT1 (DCAEVT1FILT)  encape=off
      settings: LibrarySourceBlock=c2806xlib/ePWM
  ePWM4 : c2802xlib/ePWM  PwmType=C2000  useModule=ePWM5  ePWMxLINKTBPRD=Not Linked  periodUnits=Clock cycles  timerSource=Input port  timerPeriod_clk=294  timerPeriod_sec=0.0001  tbshadow=Counter equals to zero  countingMode=Up-Down  phaseActiveEnable=Disable  phaseDirection=Count down after sync  phaseActive=0  synchronizationEnable=off  dcaevt1Sync=off  dcbevt1Sync=off  synchronizationOption=Disable  dcbevt1SyncOut=off  dcaevt1SyncOut=off  cmpdSyncOut=off  cmpcSyncOut=off  cmpbSyncOut=off  zeroSyncOut=off  swfSyncOut=off  perSynchronizationOption=Counter equals to period (CTR=PRD)  clockPrescale=1  HSclockPrescale=1  enswap=off  ePWMxAStatus=on  ePWMxAactionLogic1=Do nothing  ePWMxAactionLogic2=Do nothing  ePWMxAactionLogic3=Set  ePWMxAactionLogic4=Do nothing  ePWMxAactionLogic5=Clear  ePWMxAactionLogic6=Do nothing  ePWMxACSFenable=off  ePWMxACSFvalue=Forcing disable  ePWMxASFreload=Zero  ePWMxBStatus=on  ePWMxBactionLogic1=Do nothing  ePWMxBactionLogic2=Do nothing  ePWMxBactionLogic3=Do nothing  ePWMxBactionLogic4=Clear  ePWMxBactionLogic5=Do nothing  ePWMxBactionLogic6=Set  ePWMxBCSFenable=off  ePWMxBCSFvalue=Forcing disable  ePWMxBSFreload=Zero  ePWNxBOutWay=off  ePWMxLINKCMPA=Not Linked  CMPAUnits=Clock cycles  CMPASource=Input port  CMPAValue_per=50  CMPAValue_clk=0  enCMPAshadow=Counter equals to zero (CTR=Zero)  ePWMxLINKCMPB=Not Linked  CMPBUnits=Clock cycles  CMPBSource=Input port  CMPBValue_per=50  CMPBValue_clk=0  enCMPBshadow=Counter equals to zero (CTR=Zero)  ePWMxLINKCMPC=Not Linked  CMPCUnits=Clock cycles  CMPCSource=Specify via dialog  CMPCValue_per=50  CMPCValue_clk=32000  enCMPCshadow=Counter equals to zero (CTR=Zero)  ePWMxLINKCMPD=Not Linked  CMPDUnits=Clock cycles  CMPDSource=Specify via dialog  CMPDValue_per=50  CMPDValue_clk=32000  enCMPDshadow=Counter equals to zero (CTR=Zero)  enableDBePWMxA=off  enableDBePWMxB=off  enhalfcycle=off  DBpolarity=Active high complementary (AHC)  DBedgeDelay=Positive  DBSource_ePWMxA=ePWMxA  DBSource_ePWMxB=ePWMxA  DBPeriodUnits=Clock cycles  DBperiodSource=Input port  REDperiod=10  FEDperiod=10  REDperiod_sec=0  FEDperiod_sec=0  LoadModeDBRED=Immediate without using shadow  LoadModeDBFED=Immediate without using shadow  adcstartModuleA=on  adcrequestEventA=First event  adcstartEventA=Counter equals to zero (CTR=Zero)  adcstartEventA_type2=Digital Compare Module A Event 1 start of conversion (DCAEVT1.soc)  adcstartModuleB=off  adcrequestEventB=First event  adcstartEventB=Counter equals to zero (CTR=Zero)  adcstartEventB_type2=Counter equals to zero (CTR=Zero)  intEn=on  intPrd=First event  intSel=Counter equals to zero (CTR=Zero)  intSel_type2=Counter equals to zero (CTR=Zero)  hrpe=off  enHRPWM=off  HRPWM_LoadMode=Counter equals to period (CTR=PRD)  HRPWM_CTLMode=Duty or Period control mode  HRPWM_EDGMode=Both edge  hrpeb=off  enHRPWMB=off  HRPWM_LoadModeB=Counter equals to zero (CTR=ZERO)  HRPWM_CTLModeB=Duty or Period control mode  HRPWM_EDGModeB=Both edge  enHRDBRED=off  enHRDBFED=off  enSFO=on  enautoconv=on  chopperEnable=off  chopperFrequency=1  chopperFirstwidth=1  chopperDuty=12.5%  tripZonesource=Specify via dialog  tzselOSHT1=off  tzselOSHT2=off  tzselOSHT3=off  tzselOSHDCAEV1=off  tzselOSHDCBEV1=off  tzselCBC1=off  tzselCBC2=off  tzselCBC3=off  tzselCBCDCAEV2=off  tzselCBCDCBEV2=off  tzselOSHT4=off  tzselOSHT5=off  tzselOSHT6=off  tzselCBC4=off  tzselCBC5=off  tzselCBC6=off  enTzOstIntr=off  enTzCbcIntr=off  enTzDCAEVT1Intr=off  enTzDCAEVT2Intr=off  enTzDCBEVT1Intr=off  enTzDCBEVT2Intr=off  ePWMxAforced=No action  ePWMxBforced=No action  DCAEVT1forced=Low  DCBEVT1forced=Low  DCAEVT2forced=No action  DCBEVT2forced=No action  dcah=COMP1OUT input  dcal=Trip Zone 1 input (TZ1)  dcbh=COMP1OUT input  dcbl=Trip Zone 1 input (TZ1)  dcah_type2=GPTRIP1SEL/(TZ1)  dcal_type2=GPTRIP2SEL/(TZ2)  dcbh_type2=GPTRIP1SEL/(TZ1)  dcbl_type2=GPTRIP2SEL/(TZ2)  gendcaevt1=DCAH=high and DCAL=don't care  gendcaevt2=Event disabled  gendcbevt1=DCBH=high and DCBL=don't care  gendcbevt2=Event disabled  dcaevt1src=DCAEVT1 with sync  dcaevt2src=DCAEVT2 with sync  dcbevt1src=DCBEVT1 with sync  dcbevt2src=DCBEVT2 with sync  pulsesel=Counter equals to zero (CTR=Zero)  blankinv=off  blankoffset=0  blankwidth=0  evsrcsel=Filtered version of DCAEVT1 (DCAEVT1FILT)  encape=off
      settings: LibrarySourceBlock=c2806xlib/ePWM
  original : c2802xlib/ePWM  Commented=on  PwmType=C2000  useModule=ePWM6  ePWMxLINKTBPRD=Not Linked  periodUnits=Clock cycles  timerSource=Input port  timerPeriod_clk=294  timerPeriod_sec=0.0001  tbshadow=Counter equals to zero  countingMode=Up-Down  phaseActiveEnable=Disable  phaseDirection=Count down after sync  phaseActive=0  synchronizationEnable=off  dcaevt1Sync=off  dcbevt1Sync=off  synchronizationOption=Disable  dcbevt1SyncOut=off  dcaevt1SyncOut=off  cmpdSyncOut=off  cmpcSyncOut=off  cmpbSyncOut=off  zeroSyncOut=off  swfSyncOut=off  perSynchronizationOption=Counter equals to period (CTR=PRD)  clockPrescale=1  HSclockPrescale=1  enswap=off  ePWMxAStatus=on  ePWMxAactionLogic1=Do nothing  ePWMxAactionLogic2=Do nothing  ePWMxAactionLogic3=Set  ePWMxAactionLogic4=Do nothing  ePWMxAactionLogic5=Clear  ePWMxAactionLogic6=Do nothing  ePWMxACSFenable=off  ePWMxACSFvalue=Forcing disable  ePWMxASFreload=Zero  ePWMxBStatus=on  ePWMxBactionLogic1=Do nothing  ePWMxBactionLogic2=Do nothing  ePWMxBactionLogic3=Do nothing  ePWMxBactionLogic4=Clear  ePWMxBactionLogic5=Do nothing  ePWMxBactionLogic6=Set  ePWMxBCSFenable=off  ePWMxBCSFvalue=Forcing disable  ePWMxBSFreload=Zero  ePWNxBOutWay=off  ePWMxLINKCMPA=Not Linked  CMPAUnits=Clock cycles  CMPASource=Input port  CMPAValue_per=50  CMPAValue_clk=12  enCMPAshadow=Counter equals to zero (CTR=Zero)  ePWMxLINKCMPB=Not Linked  CMPBUnits=Clock cycles  CMPBSource=Input port  CMPBValue_per=50  CMPBValue_clk=283  enCMPBshadow=Counter equals to zero (CTR=Zero)  ePWMxLINKCMPC=Not Linked  CMPCUnits=Clock cycles  CMPCSource=Specify via dialog  CMPCValue_per=50  CMPCValue_clk=32000  enCMPCshadow=Counter equals to zero (CTR=Zero)  ePWMxLINKCMPD=Not Linked  CMPDUnits=Clock cycles  CMPDSource=Specify via dialog  CMPDValue_per=50  CMPDValue_clk=32000  enCMPDshadow=Counter equals to zero (CTR=Zero)  enableDBePWMxA=off  enableDBePWMxB=off  enhalfcycle=off  DBpolarity=Active high complementary (AHC)  DBedgeDelay=Positive  DBSource_ePWMxA=ePWMxA  DBSource_ePWMxB=ePWMxA  DBPeriodUnits=Clock cycles  DBperiodSource=Input port  REDperiod=10  FEDperiod=10  REDperiod_sec=0  FEDperiod_sec=0  LoadModeDBRED=Immediate without using shadow  LoadModeDBFED=Immediate without using shadow  adcstartModuleA=off  adcrequestEventA=First event  adcstartEventA=Counter equals to zero (CTR=Zero)  adcstartEventA_type2=Digital Compare Module A Event 1 start of conversion (DCAEVT1.soc)  adcstartModuleB=off  adcrequestEventB=First event  adcstartEventB=Counter equals to zero (CTR=Zero)  adcstartEventB_type2=Counter equals to zero (CTR=Zero)  intEn=off  intPrd=First event  intSel=Counter equals to zero (CTR=Zero)  intSel_type2=Counter equals to zero (CTR=Zero)  hrpe=off  enHRPWM=off  HRPWM_LoadMode=Counter equals to period (CTR=PRD)  HRPWM_CTLMode=Duty or Period control mode  HRPWM_EDGMode=Both edge  hrpeb=off  enHRPWMB=off  HRPWM_LoadModeB=Counter equals to zero (CTR=ZERO)  HRPWM_CTLModeB=Duty or Period control mode  HRPWM_EDGModeB=Both edge  enHRDBRED=off  enHRDBFED=off  enSFO=on  enautoconv=on  chopperEnable=off  chopperFrequency=1  chopperFirstwidth=1  chopperDuty=12.5%  tripZonesource=Specify via dialog  tzselOSHT1=off  tzselOSHT2=off  tzselOSHT3=off  tzselOSHDCAEV1=off  tzselOSHDCBEV1=off  tzselCBC1=off  tzselCBC2=off  tzselCBC3=off  tzselCBCDCAEV2=off  tzselCBCDCBEV2=off  tzselOSHT4=off  tzselOSHT5=off  tzselOSHT6=off  tzselCBC4=off  tzselCBC5=off  tzselCBC6=off  enTzOstIntr=off  enTzCbcIntr=off  enTzDCAEVT1Intr=off  enTzDCAEVT2Intr=off  enTzDCBEVT1Intr=off  enTzDCBEVT2Intr=off  ePWMxAforced=No action  ePWMxBforced=No action  DCAEVT1forced=Low  DCBEVT1forced=Low  DCAEVT2forced=No action  DCBEVT2forced=No action  dcah=COMP1OUT input  dcal=Trip Zone 1 input (TZ1)  dcbh=COMP1OUT input  dcbl=Trip Zone 1 input (TZ1)  dcah_type2=GPTRIP1SEL/(TZ1)  dcal_type2=GPTRIP2SEL/(TZ2)  dcbh_type2=GPTRIP1SEL/(TZ1)  dcbl_type2=GPTRIP2SEL/(TZ2)  gendcaevt1=DCAH=high and DCAL=don't care  gendcaevt2=Event disabled  gendcbevt1=DCBH=high and DCBL=don't care  gendcbevt2=Event disabled  dcaevt1src=DCAEVT1 with sync  dcaevt2src=DCAEVT2 with sync  dcbevt1src=DCBEVT1 with sync  dcbevt2src=DCBEVT2 with sync  pulsesel=Counter equals to zero (CTR=Zero)  blankinv=off  blankoffset=0  blankwidth=0  evsrcsel=Filtered version of DCAEVT1 (DCAEVT1FILT)  encape=off
      settings: LibrarySourceBlock=c2806xlib/ePWM
  u : ArgIn  DisableCoverage=on  ArgumentName=u
  u1 : ArgIn  DisableCoverage=on  Port=2  OutDataTypeStr=uint16  ArgumentName=u1
  wires:
  Gain/1 -> Floor/1
  Constant3/1 -> Subsystem1/2(Duty(%))
  Gain2/1 -> Divide/1, Dead time (%)/1
  Product1/1 -> Gain2/1
  u1/1 -> Product1/3
  Constant4/1 -> Switch1/3
  Product4/1 -> CMPB1/1, ePWM1/3, ePWM4/3
  Product3/1 -> CMPA1/1, ePWM4/2, ePWM1/2
  Switch/1 -> Product4/2, Product3/2
  Constant2/1 -> Switch/3
  Constant1/1 -> Switch/1
  Dead time (sec)/1 -> Product1/2
  Gain1/1 -> Product1/1
  Floor/1 -> ePWM1/1, ePWM4/1, Subtract/1, Product2/1
  Subtract/1 -> CMPB/1, Product4/1
  Constant/1 -> Divide/2
  Product2/1 -> CMPA/1, Product3/1, Subtract/2
  Divide/1 -> Product2/2
  u/1 -> Switch1/2, Switch1/1
  Switch1/1 -> Gain1/1, Switch/2, Gain/1
